simulink model "whileloop"  (R2021a)
settings: Solver=FixedStepDiscrete  StartTime=0.0  StopTime=10.0  RelTol=1e-3
settings Model: Creator=LEGION  LastModifiedBy=LEGION
settings OptimizationCC: DefaultParameterBehavior=Inlined  EnhancedBackFolding=on  PassReuseOutputArgsAs=Individual arguments  ZeroExternalMemoryAtStartup=off  ZeroInternalMemoryAtStartup=off  OptimizeBlockOrder=speed  DifferentSizesBufferReuse=on  OptimizationCustomize=off  EfficientTunableParamExpr=on
settings DebuggingCC: ParameterTunabilityLossMsg=error
settings SFSimCC: MATLABDynamicMemAlloc=off
settings RTWCC: SystemTargetFile=ert.tlc  GenCodeOnly=on  TemplateMakefile=ert_default_tmf  GenerateReport=on  IncludeHyperlinkInReport=on  LaunchReport=on  GenerateTraceInfo=on
settings CodeAppCC: ForceParamTrailComments=on  IgnoreCustomStorageClasses=off  OperatorAnnotations=on  SimulinkDataObjDesc=on  SFDataObjDesc=on  InsertBlockDesc=on
settings ERTTargetCC: TargetLangStandard=C99 (ISO)  GenerateSampleERTMain=on  InlinedParameterPlacement=NonHierarchical  ERTCustomFileTemplate=example_file_process.tlc  EnableUserReplacementTypes=on

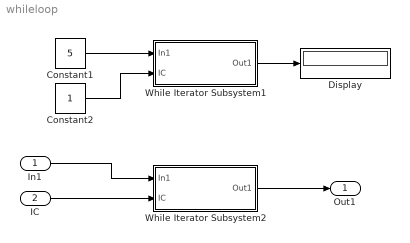
== system whileloop ==
  In1 : Inport
  IC : Inport  Port=2
  Constant1 : Constant  Value=5
  Constant2 : Constant
  Display : Display
  While Iterator Subsystem1 : Subsystem  TreatAsAtomicUnit=on
  While Iterator Subsystem2 : Subsystem  TreatAsAtomicUnit=on
  Out1 : Outport
  wires:
  IC/1 -> While Iterator Subsystem2/2(IC)
  In1/1 -> While Iterator Subsystem2/1(In1)
  Constant1/1 -> While Iterator Subsystem1/1(In1)
  Constant2/1 -> While Iterator Subsystem1/2(IC)
  While Iterator Subsystem1/1(Out1) -> Display/1
  While Iterator Subsystem2/1(Out1) -> Out1/1

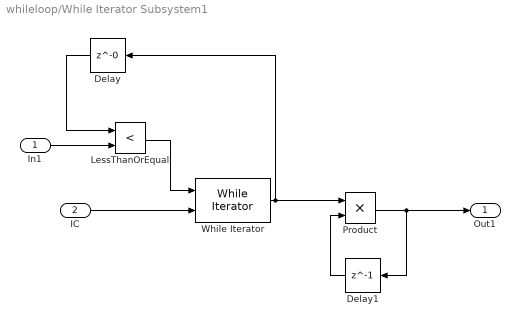
== system whileloop/While Iterator Subsystem1 ==
  In1 : Inport
  IC : Inport  Port=2
  Delay : Delay  DelayLength=0  InitialCondition=0
  Delay1 : Delay  DelayLength=1  InitialCondition=1
  LessThanOrEqual : RelationalOperator  Operator=<  OutDataTypeStr=boolean  RndMeth=Simplest
  Product : Product  OutDataTypeStr=int32
  While Iterator : WhileIterator  MaxIters=-1  ShowIterationPort=on
  Out1 : Outport  OutDataTypeStr=int32
  wires:
  IC/1 -> While Iterator/2
  LessThanOrEqual/1 -> While Iterator/1
  In1/1 -> LessThanOrEqual/2
  Delay/1 -> LessThanOrEqual/1
  Product/1 -> Delay1/1, Out1/1
  Delay1/1 -> Product/2
  While Iterator/1 -> Delay/1, Product/1

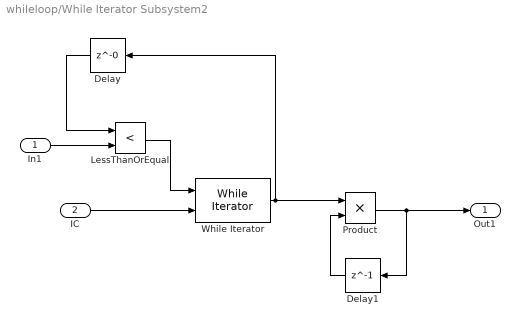
== system whileloop/While Iterator Subsystem2 ==
  In1 : Inport
  IC : Inport  Port=2
  Delay : Delay  DelayLength=0  InitialCondition=0
  Delay1 : Delay  DelayLength=1  InitialCondition=1
  LessThanOrEqual : RelationalOperator  Operator=<  OutDataTypeStr=boolean  RndMeth=Simplest
  Product : Product  OutDataTypeStr=int32
  While Iterator : WhileIterator  MaxIters=-1  ShowIterationPort=on
  Out1 : Outport  OutDataTypeStr=int32
  wires:
  IC/1 -> While Iterator/2
  LessThanOrEqual/1 -> While Iterator/1
  In1/1 -> LessThanOrEqual/2
  Delay/1 -> LessThanOrEqual/1
  Product/1 -> Delay1/1, Out1/1
  Delay1/1 -> Product/2
  While Iterator/1 -> Delay/1, Product/1
